simulink model "e8_lookuptable_NN_cex"  (R2020a)
settings: Solver=FixedStepDiscrete  StartTime=0.0  StopTime=options.T_train  RelTol=1e-3
PreLoadFcn:
  | Ts = 0.1;
  | Plant = c2d(zpk([],[-1 -3 -5],1),Ts);
  | C0 = pid(1,1,1,'Ts',Ts,'IF','B','DF','B'); % define PID structure
  | C = pidtune(Plant,C0); % design PID
  | [Kp Ki Kd] = piddata(C); % obtain PID gains
  | FIS = sugfis;
  | FIS = addInput(FIS,[-10 10],'Name','E');
  | FIS = addMF(FIS,'E','gaussmf',[7 -10],'Name','Negative');
  | FIS = addMF(FIS,'E','gaussmf',[7 10],'Name','Positive');
  | FIS = addInput(FIS,[-10 10],'Name','CE');
  | FIS = addMF(FIS,'CE','gaussmf',[7 -10],'Name','Negative');
  | FIS = addMF(FIS,'CE','gaussmf',[7 10],'Name','Positive');
  | FIS = addOutput(FIS,[-20 20],'Name','u');
  | FIS = addMF(FIS,'u','constant',-20,'Name','Min');
  | FIS = addMF(FIS,'u','constant',0,'Name','Zero');
  | FIS = addMF(FIS,'u','constant',20,'Name','Max');
  | ruleList = [1 1 1 1 1;...   % Rule 1
  |             1 2 2 1 1;...   % Rule 2
  |             2 1 2 1 1;...   % Rule 3
  |             2 2 3 1 1];     % Rule 4
  | FIS = addRule(FIS,ruleList);GE = 10;
  | GCE = GE*(Kp-sqrt(Kp^2-4*Ki*Kd))/2/Ki;
  | GCU = Ki/GE;
  | GU = Kd/GCE;
  | Step = 1; % use 21 break points for both E and CE inputs
  | E = -10:Step:10;
  | CE = -10:Step:10;
  | N = length(E);
  | LookUpTableData = zeros(N);
  | for i=1:N
  |    for j=1:N
  |       % compute output u for each combination of break points
  |       LookUpTableData(i,j) = evalfis(FIS,[E(i) CE(j)]);
  |    end
  | end
values from neighbouring files (symbols this model uses):
  Kd = 9.02059569264    [e8_initialize.mat]
  Ki = 25.1789147864    [e8_initialize.mat]
  Kp = 30.6494706477    [e8_initialize.mat]
undefined symbols (not defined in the file or in its folder): DiscIntNeverNeededParam, options
libraries: neural x50, cstblocks x3, simulink x2
(part 2 of 2)

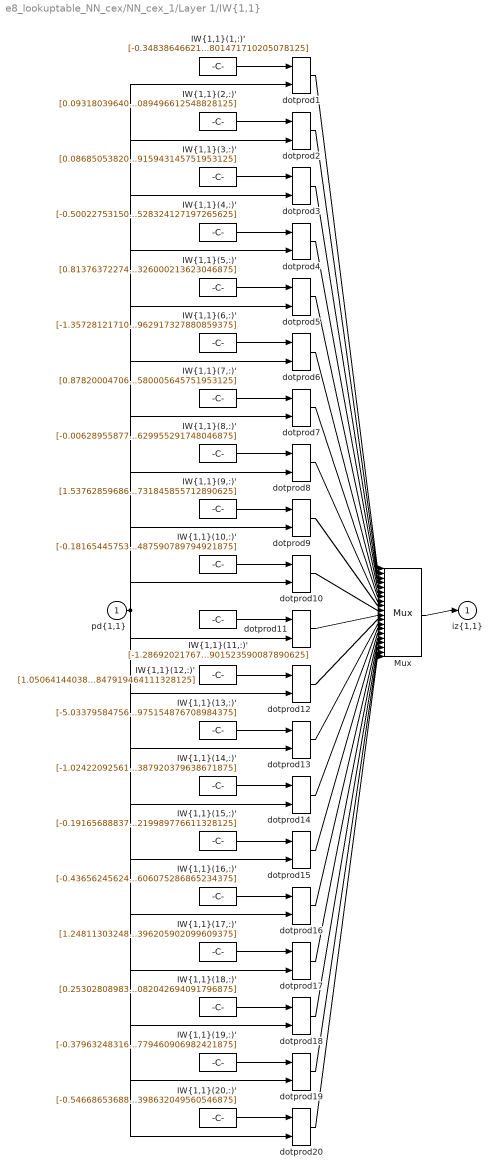
== system e8_lookuptable_NN_cex/NN_cex_1/Layer 1/IW{1,1} ==
  "pd{1,1}" : Inport  PortDimensions=6
      mask Display: e = 0.06;c1 = [120 230 180]/255;c2 = ([120 230 180]+0)/(256+128);c3 = ([120 230 180]+128)/(256+128);patch([0 1 1 0],[0 0 1 1],c1);patch([0 1 1 1-e 1-e 0+e],[0 0 1 1-e 0+e 0+e],c2);patch([0 0 1 1-e 0+e 0+e],[0 1 1 1-e 1-e 0+e],c3);plot([0 1 1 0 0],[0 0 1 1 0]);
  "IW{1,1}(1,:)'" : Constant  Value=[-0.348386466219023527290943320622318424284458160400390625;0.1425394664908231912026082000011228956282138824462890625;-0.556378117908738811792090928065590560436248779296875;2.730357611772159742713483865372836589813232421875;3.1137652539351154956648315419442951679229736328125;-3.027586211689758943776951127802021801471710205078125]
      mask Display: e = 0.06;c1 = [120 150 230]/255;c2 = ([120 150 230]+0)/383;c3 = ([120 150 230]+128)/383;patch([0 1 1 0],[0 0 1 1],c1);patch([0 1 1 1-e 1-e 0+e],[0 0 1 1-e 0+e 0+e],c2);patch([0 0 1 1-e 0+e 0+e],[0 1 1 1-e 1-e 0+e],c3);plot([0 1 1 0 0],[0 0 1 1 0]);disp('Weights');
  "IW{1,1}(10,:)'" : Constant  Value=[-0.1816544575334319844284181044713477604091167449951171875;0.055806105686074268523721997325992560945451259613037109375;0.2611160045754055136768556621973402798175811767578125;-1.399614859678795397712747217155992984771728515625;2.2935772550968778205060516484081745147705078125;-1.2593650044780424490653558677877299487590789794921875]
      mask Display: e = 0.06;c1 = [120 150 230]/255;c2 = ([120 150 230]+0)/383;c3 = ([120 150 230]+128)/383;patch([0 1 1 0],[0 0 1 1],c1);patch([0 1 1 1-e 1-e 0+e],[0 0 1 1-e 0+e 0+e],c2);patch([0 0 1 1-e 0+e 0+e],[0 1 1 1-e 1-e 0+e],c3);plot([0 1 1 0 0],[0 0 1 1 0]);disp('Weights');
  "IW{1,1}(11,:)'" : Constant  Value=[-1.286920217674374367078371506067924201488494873046875;-2.609581766566260174755598200135864317417144775390625;-5.17083618286434187893974012695252895355224609375;3.818297784345167311670365961617790162563323974609375;2.923291438037872946864581535919569432735443115234375;2.50047149548030489540906273759901523590087890625]
      mask Display: e = 0.06;c1 = [120 150 230]/255;c2 = ([120 150 230]+0)/383;c3 = ([120 150 230]+128)/383;patch([0 1 1 0],[0 0 1 1],c1);patch([0 1 1 1-e 1-e 0+e],[0 0 1 1-e 0+e 0+e],c2);patch([0 0 1 1-e 0+e 0+e],[0 1 1 1-e 1-e 0+e],c3);plot([0 1 1 0 0],[0 0 1 1 0]);disp('Weights');
  "IW{1,1}(12,:)'" : Constant  Value=[1.0506414403852952776929896572255529463291168212890625;0.446232100600356396125079072589869610965251922607421875;1.0660394205350616214644787760335020720958709716796875;0.0948846128429960133932041799198486842215061187744140625;0.92813972695216973018972339559695683419704437255859375;-0.377169606776960097960227358271367847919464111328125]
      mask Display: e = 0.06;c1 = [120 150 230]/255;c2 = ([120 150 230]+0)/383;c3 = ([120 150 230]+128)/383;patch([0 1 1 0],[0 0 1 1],c1);patch([0 1 1 1-e 1-e 0+e],[0 0 1 1-e 0+e 0+e],c2);patch([0 0 1 1-e 0+e 0+e],[0 1 1 1-e 1-e 0+e],c3);plot([0 1 1 0 0],[0 0 1 1 0]);disp('Weights');
  "IW{1,1}(13,:)'" : Constant  Value=[-5.0337958475624819953964106389321386814117431640625;-0.567401670277573710876595214358530938625335693359375;2.3534561662445749874450484639964997768402099609375;1.408344788625278898308579300646670162677764892578125;1.3822950845649817352978061535395681858062744140625;0.69787032458982822813453594790189526975154876708984375]
      mask Display: e = 0.06;c1 = [120 150 230]/255;c2 = ([120 150 230]+0)/383;c3 = ([120 150 230]+128)/383;patch([0 1 1 0],[0 0 1 1],c1);patch([0 1 1 1-e 1-e 0+e],[0 0 1 1-e 0+e 0+e],c2);patch([0 0 1 1-e 0+e 0+e],[0 1 1 1-e 1-e 0+e],c3);plot([0 1 1 0 0],[0 0 1 1 0]);disp('Weights');
  "IW{1,1}(14,:)'" : Constant  Value=[-1.0242209256128174121869278678786940872669219970703125;-2.2937759783651170408802499878220260143280029296875;-4.64904686530471966676714146160520613193511962890625;1.7028354610183387141120192609378136694431304931640625;4.84827066866913281018014458823017776012420654296875;1.5575389657167277857041653987835161387920379638671875]
      mask Display: e = 0.06;c1 = [120 150 230]/255;c2 = ([120 150 230]+0)/383;c3 = ([120 150 230]+128)/383;patch([0 1 1 0],[0 0 1 1],c1);patch([0 1 1 1-e 1-e 0+e],[0 0 1 1-e 0+e 0+e],c2);patch([0 0 1 1-e 0+e 0+e],[0 1 1 1-e 1-e 0+e],c3);plot([0 1 1 0 0],[0 0 1 1 0]);disp('Weights');
  "IW{1,1}(15,:)'" : Constant  Value=[-0.1916568883758186514487675822238088585436344146728515625;-0.955536837924347626227472574100829660892486572265625;1.7640840012597378549941140590817667543888092041015625;-6.2627507808460958216301150969229638576507568359375;3.31945471130751457167207263410091400146484375;1.695917564409768818478596585919149219989776611328125]
      mask Display: e = 0.06;c1 = [120 150 230]/255;c2 = ([120 150 230]+0)/383;c3 = ([120 150 230]+128)/383;patch([0 1 1 0],[0 0 1 1],c1);patch([0 1 1 1-e 1-e 0+e],[0 0 1 1-e 0+e 0+e],c2);patch([0 0 1 1-e 0+e 0+e],[0 1 1 1-e 1-e 0+e],c3);plot([0 1 1 0 0],[0 0 1 1 0]);disp('Weights');
  "IW{1,1}(16,:)'" : Constant  Value=[-0.436562456245822849698612344582215882837772369384765625;-0.58807402799713137664383566516335122287273406982421875;0.62844101399535612362257097629480995237827301025390625;-3.392368638141128212026842447812668979167938232421875;0.717895602299947643842870093067176640033721923828125;2.24231790817705611829069312079809606075286865234375]
      mask Display: e = 0.06;c1 = [120 150 230]/255;c2 = ([120 150 230]+0)/383;c3 = ([120 150 230]+128)/383;patch([0 1 1 0],[0 0 1 1],c1);patch([0 1 1 1-e 1-e 0+e],[0 0 1 1-e 0+e 0+e],c2);patch([0 0 1 1-e 0+e 0+e],[0 1 1 1-e 1-e 0+e],c3);plot([0 1 1 0 0],[0 0 1 1 0]);disp('Weights');
  "IW{1,1}(17,:)'" : Constant  Value=[1.248113032481268813711494658491574227809906005859375;2.902154819437817057092843242571689188480377197265625;5.286528812965197943185557960532605648040771484375;-3.243808383183388599491081549786031246185302734375;-0.755141475203453094167116432799957692623138427734375;-5.6171666528945110030690557323396205902099609375]
      mask Display: e = 0.06;c1 = [120 150 230]/255;c2 = ([120 150 230]+0)/383;c3 = ([120 150 230]+128)/383;patch([0 1 1 0],[0 0 1 1],c1);patch([0 1 1 1-e 1-e 0+e],[0 0 1 1-e 0+e 0+e],c2);patch([0 0 1 1-e 0+e 0+e],[0 1 1 1-e 1-e 0+e],c3);plot([0 1 1 0 0],[0 0 1 1 0]);disp('Weights');
  "IW{1,1}(18,:)'" : Constant  Value=[0.253028089839262670945885247419937513768672943115234375;-0.569037790042783431232464863569475710391998291015625;-2.87075007378417712544660389539785683155059814453125;0.1846358903926413608242995678665465675294399261474609375;0.97185979099097730138367978725000284612178802490234375;2.088738493855760491868522876757197082042694091796875]
      mask Display: e = 0.06;c1 = [120 150 230]/255;c2 = ([120 150 230]+0)/383;c3 = ([120 150 230]+128)/383;patch([0 1 1 0],[0 0 1 1],c1);patch([0 1 1 1-e 1-e 0+e],[0 0 1 1-e 0+e 0+e],c2);patch([0 0 1 1-e 0+e 0+e],[0 1 1 1-e 1-e 0+e],c3);plot([0 1 1 0 0],[0 0 1 1 0]);disp('Weights');
  "IW{1,1}(19,:)'" : Constant  Value=[-0.379632483162776368512680846833973191678524017333984375;-1.823585261164791138099872114253230392932891845703125;1.7068136710403318812012685157242231070995330810546875;-1.155374696821884317188278146204538643360137939453125;-2.390442322815810261005253778421320021152496337890625;0.11907895833631725046597438222306664101779460906982421875]
      mask Display: e = 0.06;c1 = [120 150 230]/255;c2 = ([120 150 230]+0)/383;c3 = ([120 150 230]+128)/383;patch([0 1 1 0],[0 0 1 1],c1);patch([0 1 1 1-e 1-e 0+e],[0 0 1 1-e 0+e 0+e],c2);patch([0 0 1 1-e 0+e 0+e],[0 1 1 1-e 1-e 0+e],c3);plot([0 1 1 0 0],[0 0 1 1 0]);disp('Weights');
  "IW{1,1}(2,:)'" : Constant  Value=[0.09318039640996118866400621527645853348076343536376953125;2.079305273090553907167077341000549495220184326171875;4.464104951807509991112965508364140987396240234375;-1.05937005318864319036720189615152776241302490234375;0.06508701563954789881538687268403009511530399322509765625;-2.682738056224437617203193440218456089496612548828125]
      mask Display: e = 0.06;c1 = [120 150 230]/255;c2 = ([120 150 230]+0)/383;c3 = ([120 150 230]+128)/383;patch([0 1 1 0],[0 0 1 1],c1);patch([0 1 1 1-e 1-e 0+e],[0 0 1 1-e 0+e 0+e],c2);patch([0 0 1 1-e 0+e 0+e],[0 1 1 1-e 1-e 0+e],c3);plot([0 1 1 0 0],[0 0 1 1 0]);disp('Weights');
  "IW{1,1}(20,:)'" : Constant  Value=[-0.54668653688684820668441943780635483562946319580078125;0.71502457693553489459503680336638353765010833740234375;-5.43924005346282424255832665949128568172454833984375;4.68030196116046948162647822755388915538787841796875;1.8413784503064121178539380707661621272563934326171875;-1.1292548199595369151637669347110204398632049560546875]
      mask Display: e = 0.06;c1 = [120 150 230]/255;c2 = ([120 150 230]+0)/383;c3 = ([120 150 230]+128)/383;patch([0 1 1 0],[0 0 1 1],c1);patch([0 1 1 1-e 1-e 0+e],[0 0 1 1-e 0+e 0+e],c2);patch([0 0 1 1-e 0+e 0+e],[0 1 1 1-e 1-e 0+e],c3);plot([0 1 1 0 0],[0 0 1 1 0]);disp('Weights');
  "IW{1,1}(3,:)'" : Constant  Value=[0.0868505382045303975235839288870920427143573760986328125;1.8533625624952818622404038251261226832866668701171875;4.0910317499985584532851135008968412876129150390625;0.203963661141593088910184405904146842658519744873046875;-2.140980212086158740447672244044952094554901123046875;-1.2946799838017259975941897209850139915943145751953125]
      mask Display: e = 0.06;c1 = [120 150 230]/255;c2 = ([120 150 230]+0)/383;c3 = ([120 150 230]+128)/383;patch([0 1 1 0],[0 0 1 1],c1);patch([0 1 1 1-e 1-e 0+e],[0 0 1 1-e 0+e 0+e],c2);patch([0 0 1 1-e 0+e 0+e],[0 1 1 1-e 1-e 0+e],c3);plot([0 1 1 0 0],[0 0 1 1 0]);disp('Weights');
  "IW{1,1}(4,:)'" : Constant  Value=[-0.50022753150170073954683402916998602449893951416015625;0.52395148428176108179599168579443357884883880615234375;-0.2282564379463638826184279650988173671066761016845703125;-0.216668457662572311317461526414263062179088592529296875;0.74276123834498253284408519903081469237804412841796875;-0.7843545765266333180676383562968112528324127197265625]
      mask Display: e = 0.06;c1 = [120 150 230]/255;c2 = ([120 150 230]+0)/383;c3 = ([120 150 230]+128)/383;patch([0 1 1 0],[0 0 1 1],c1);patch([0 1 1 1-e 1-e 0+e],[0 0 1 1-e 0+e 0+e],c2);patch([0 0 1 1-e 0+e 0+e],[0 1 1 1-e 1-e 0+e],c3);plot([0 1 1 0 0],[0 0 1 1 0]);disp('Weights');
  "IW{1,1}(5,:)'" : Constant  Value=[0.813763722741680961547672268352471292018890380859375;-1.26725708973505657439773131045512855052947998046875;1.05747593097696057640177969005890190601348876953125;4.017914528050038569517710129730403423309326171875;-1.00458918139684261205957227502949535846710205078125;-3.59420075961118623553147699567489326000213623046875]
      mask Display: e = 0.06;c1 = [120 150 230]/255;c2 = ([120 150 230]+0)/383;c3 = ([120 150 230]+128)/383;patch([0 1 1 0],[0 0 1 1],c1);patch([0 1 1 1-e 1-e 0+e],[0 0 1 1-e 0+e 0+e],c2);patch([0 0 1 1-e 0+e 0+e],[0 1 1 1-e 1-e 0+e],c3);plot([0 1 1 0 0],[0 0 1 1 0]);disp('Weights');
  "IW{1,1}(6,:)'" : Constant  Value=[-1.3572812171043395768066375239868648350238800048828125;-0.807843543346363102131135747185908257961273193359375;-1.52364712049379047442698720260523259639739990234375;0.01055194339140820558586852939697564579546451568603515625;-0.178172231604927178150177269344567321240901947021484375;2.1452691178145126826848354539833962917327880859375]
      mask Display: e = 0.06;c1 = [120 150 230]/255;c2 = ([120 150 230]+0)/383;c3 = ([120 150 230]+128)/383;patch([0 1 1 0],[0 0 1 1],c1);patch([0 1 1 1-e 1-e 0+e],[0 0 1 1-e 0+e 0+e],c2);patch([0 0 1 1-e 0+e 0+e],[0 1 1 1-e 1-e 0+e],c3);plot([0 1 1 0 0],[0 0 1 1 0]);disp('Weights');
  "IW{1,1}(7,:)'" : Constant  Value=[0.8782000470625199728402776599978096783161163330078125;2.18085604374191976972952033975161612033843994140625;3.68222221341653721538023091852664947509765625;-0.7144715143483979513661097371368668973445892333984375;-3.67514376155449529193219859735108911991119384765625;-5.52543277574851021682889040675945580005645751953125]
      mask Display: e = 0.06;c1 = [120 150 230]/255;c2 = ([120 150 230]+0)/383;c3 = ([120 150 230]+128)/383;patch([0 1 1 0],[0 0 1 1],c1);patch([0 1 1 1-e 1-e 0+e],[0 0 1 1-e 0+e 0+e],c2);patch([0 0 1 1-e 0+e 0+e],[0 1 1 1-e 1-e 0+e],c3);plot([0 1 1 0 0],[0 0 1 1 0]);disp('Weights');
  "IW{1,1}(8,:)'" : Constant  Value=[-0.0062895587781400530413833394050016067922115325927734375;2.0813121464876207511451866594143211841583251953125;1.41298158685531660694323363713920116424560546875;2.610797383555816253419834538362920284271240234375;-2.934393295729890827061581148882396519184112548828125;-3.211793760885452098108316931757144629955291748046875]
      mask Display: e = 0.06;c1 = [120 150 230]/255;c2 = ([120 150 230]+0)/383;c3 = ([120 150 230]+128)/383;patch([0 1 1 0],[0 0 1 1],c1);patch([0 1 1 1-e 1-e 0+e],[0 0 1 1-e 0+e 0+e],c2);patch([0 0 1 1-e 0+e 0+e],[0 1 1 1-e 1-e 0+e],c3);plot([0 1 1 0 0],[0 0 1 1 0]);disp('Weights');
  "IW{1,1}(9,:)'" : Constant  Value=[1.5376285968624461286680116245406679809093475341796875;3.460302608257689538362456005415879189968109130859375;5.632796285788128187732581864111125469207763671875;-3.38287395323599060503738655825145542621612548828125;-2.347627611400820768494668300263583660125732421875;-5.1162623231328101525150486850179731845855712890625]
      mask Display: e = 0.06;c1 = [120 150 230]/255;c2 = ([120 150 230]+0)/383;c3 = ([120 150 230]+128)/383;patch([0 1 1 0],[0 0 1 1],c1);patch([0 1 1 1-e 1-e 0+e],[0 0 1 1-e 0+e 0+e],c2);patch([0 0 1 1-e 0+e 0+e],[0 1 1 1-e 1-e 0+e],c3);plot([0 1 1 0 0],[0 0 1 1 0]);disp('Weights');
  Mux : Mux  Inputs=20
      mask Display: e = 0.06;c1 = [120 150 230]/255;c2 = ([120 150 230]+0)/383;c3 = ([120 150 230]+128)/383;patch([0 1 1 0],[0 0 1 1],c1);patch([0 1 1 1-e 1-e 0+e],[0 0 1 1-e 0+e 0+e],c2);patch([0 0 1 1-e 0+e 0+e],[0 1 1 1-e 1-e 0+e],c3);plot([0 1 1 0 0],[0 0 1 1 0]);disp('Mux');
  dotprod{1..20} (20 alike) : neural/Weight Functions/dotprod
  "iz{1,1}" : Outport
      mask Display: e = 0.06;c1 = [120 230 180]/255;c2 = ([120 230 180]+0)/(256+128);c3 = ([120 230 180]+128)/(256+128);patch([0 1 1 0],[0 0 1 1],c1);patch([0 1 1 1-e 1-e 0+e],[0 0 1 1-e 0+e 0+e],c2);patch([0 0 1 1-e 0+e 0+e],[0 1 1 1-e 1-e 0+e],c3);plot([0 1 1 0 0],[0 0 1 1 0]);
  wires:
  "IW{1,1}(1,:)'"/1 -> dotprod1/1
  "pd{1,1}"/1 -> dotprod1/2, dotprod2/2, dotprod3/2, dotprod4/2, dotprod5/2, dotprod6/2, dotprod7/2, dotprod8/2, dotprod9/2, dotprod10/2, dotprod11/2, dotprod12/2, dotprod13/2, dotprod14/2, dotprod15/2, dotprod16/2, dotprod17/2, dotprod18/2, dotprod19/2, dotprod20/2
  dotprod1/1 -> Mux/1
  "IW{1,1}(2,:)'"/1 -> dotprod2/1
  dotprod2/1 -> Mux/2
  "IW{1,1}(3,:)'"/1 -> dotprod3/1
  dotprod3/1 -> Mux/3
  "IW{1,1}(4,:)'"/1 -> dotprod4/1
  dotprod4/1 -> Mux/4
  "IW{1,1}(5,:)'"/1 -> dotprod5/1
  dotprod5/1 -> Mux/5
  "IW{1,1}(6,:)'"/1 -> dotprod6/1
  dotprod6/1 -> Mux/6
  "IW{1,1}(7,:)'"/1 -> dotprod7/1
  dotprod7/1 -> Mux/7
  "IW{1,1}(8,:)'"/1 -> dotprod8/1
  dotprod8/1 -> Mux/8
  "IW{1,1}(9,:)'"/1 -> dotprod9/1
  dotprod9/1 -> Mux/9
  "IW{1,1}(10,:)'"/1 -> dotprod10/1
  dotprod10/1 -> Mux/10
  "IW{1,1}(11,:)'"/1 -> dotprod11/1
  dotprod11/1 -> Mux/11
  "IW{1,1}(12,:)'"/1 -> dotprod12/1
  dotprod12/1 -> Mux/12
  "IW{1,1}(13,:)'"/1 -> dotprod13/1
  dotprod13/1 -> Mux/13
  "IW{1,1}(14,:)'"/1 -> dotprod14/1
  dotprod14/1 -> Mux/14
  "IW{1,1}(15,:)'"/1 -> dotprod15/1
  dotprod15/1 -> Mux/15
  "IW{1,1}(16,:)'"/1 -> dotprod16/1
  dotprod16/1 -> Mux/16
  "IW{1,1}(17,:)'"/1 -> dotprod17/1
  dotprod17/1 -> Mux/17
  "IW{1,1}(18,:)'"/1 -> dotprod18/1
  dotprod18/1 -> Mux/18
  "IW{1,1}(19,:)'"/1 -> dotprod19/1
  dotprod19/1 -> Mux/19
  "IW{1,1}(20,:)'"/1 -> dotprod20/1
  dotprod20/1 -> Mux/20
  Mux/1 -> "iz{1,1}"/1

== system e8_lookuptable_NN_cex/NN_cex_1/Layer 2/Delays 1 ==
  "p{2}" : Inport  PortDimensions=20
      mask Display: e = 0.06;c1 = [120 230 180]/255;c2 = ([120 230 180]+0)/(256+128);c3 = ([120 230 180]+128)/(256+128);patch([0 1 1 0],[0 0 1 1],c1);patch([0 1 1 1-e 1-e 0+e],[0 0 1 1-e 0+e 0+e],c2);patch([0 0 1 1-e 0+e 0+e],[0 1 1 1-e 1-e 0+e],c3);plot([0 1 1 0 0],[0 0 1 1 0]);
  mux : Mux  Inputs=1
      mask Display: e = 0.06;c1 = [120 150 230]/255;c2 = ([120 150 230]+0)/383;c3 = ([120 150 230]+128)/383;patch([0 1 1 0],[0 0 1 1],c1);patch([0 1 1 1-e 1-e 0+e],[0 0 1 1-e 0+e 0+e],c2);patch([0 0 1 1-e 0+e 0+e],[0 1 1 1-e 1-e 0+e],c3);plot([0 1 1 0 0],[0 0 1 1 0]);disp('Mux')
  "pd{2,1}" : Outport
      mask Display: e = 0.06;c1 = [120 230 180]/255;c2 = ([120 230 180]+0)/(256+128);c3 = ([120 230 180]+128)/(256+128);patch([0 1 1 0],[0 0 1 1],c1);patch([0 1 1 1-e 1-e 0+e],[0 0 1 1-e 0+e 0+e],c2);patch([0 0 1 1-e 0+e 0+e],[0 1 1 1-e 1-e 0+e],c3);plot([0 1 1 0 0],[0 0 1 1 0]);
  wires:
  "p{2}"/1 -> mux/1
  mux/1 -> "pd{2,1}"/1

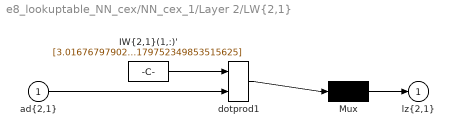
== system e8_lookuptable_NN_cex/NN_cex_1/Layer 2/LW{2,1} ==
  "ad{2,1}" : Inport  PortDimensions=20
      mask Display: e = 0.06;c1 = [120 230 180]/255;c2 = ([120 230 180]+0)/(256+128);c3 = ([120 230 180]+128)/(256+128);patch([0 1 1 0],[0 0 1 1],c1);patch([0 1 1 1-e 1-e 0+e],[0 0 1 1-e 0+e 0+e],c2);patch([0 0 1 1-e 0+e 0+e],[0 1 1 1-e 1-e 0+e],c3);plot([0 1 1 0 0],[0 0 1 1 0]);
  "IW{2,1}(1,:)'" : Constant  Value=[3.01676797902892968039623156073503196239471435546875;1.32346425952183466279166168533265590667724609375;-1.5287563496158593778773138183169066905975341796875;-1.9425943597265964424281037281616590917110443115234375;1.0693673842509243687715070336707867681980133056640625;0.07552468599520467673613666192977689206600189208984375;-0.01435443552857789718812941970327301532961428165435791015625;-3.65419260335727091870694493991322815418243408203125;-1.7836352235567434210139481365331448614597320556640625;-2.472390499067472990901705998112447559833526611328125;-3.37090558998205924723379212082363665103912353515625;0.16030133524802103739403946747188456356525421142578125;-0.376330459121932248134356768787256442010402679443359375;-2.89732175648036704984633615822531282901763916015625;3.12621113122824478836037087603472173213958740234375;0.73662093394306449312125550932250916957855224609375;-1.2532743301873903174481483802082948386669158935546875;-4.1653477500658571130998097942210733890533447265625;0.0544208934024130730477963879820890724658966064453125;3.34664442605948497799772667349316179752349853515625]
      mask Display: e = 0.06;c1 = [120 150 230]/255;c2 = ([120 150 230]+0)/383;c3 = ([120 150 230]+128)/383;patch([0 1 1 0],[0 0 1 1],c1);patch([0 1 1 1-e 1-e 0+e],[0 0 1 1-e 0+e 0+e],c2);patch([0 0 1 1-e 0+e 0+e],[0 1 1 1-e 1-e 0+e],c3);plot([0 1 1 0 0],[0 0 1 1 0]);disp('weights');
  Mux : Mux  Inputs=1
      mask Display: e = 0.06;c1 = [120 150 230]/255;c2 = ([120 150 230]+0)/383;c3 = ([120 150 230]+128)/383;patch([0 1 1 0],[0 0 1 1],c1);patch([0 1 1 1-e 1-e 0+e],[0 0 1 1-e 0+e 0+e],c2);patch([0 0 1 1-e 0+e 0+e],[0 1 1 1-e 1-e 0+e],c3);plot([0 1 1 0 0],[0 0 1 1 0]);disp('Mux');
  dotprod1 : neural/Weight Functions/dotprod
  "lz{2,1}" : Outport
      mask Display: e = 0.06;c1 = [120 230 180]/255;c2 = ([120 230 180]+0)/(256+128);c3 = ([120 230 180]+128)/(256+128);patch([0 1 1 0],[0 0 1 1],c1);patch([0 1 1 1-e 1-e 0+e],[0 0 1 1-e 0+e 0+e],c2);patch([0 0 1 1-e 0+e 0+e],[0 1 1 1-e 1-e 0+e],c3);plot([0 1 1 0 0],[0 0 1 1 0]);
  wires:
  "IW{2,1}(1,:)'"/1 -> dotprod1/1
  "ad{2,1}"/1 -> dotprod1/2
  dotprod1/1 -> Mux/1
  Mux/1 -> "lz{2,1}"/1
